simulink model "q_sip_lqr_q8_ip02"  (Simulink 4.00)
settings: Solver=ode4  SolverMode=SingleTasking  StartTime=0.0  StopTime=9999  FixedStep=0.001  RelTol=1e-3  AbsTol=1e-6
values from neighbouring files (symbols this model uses):
  C = eye( 4 )    [d_ip01_2_sip_lqr.m]
  D = zeros( 4, 1 )    [d_ip01_2_sip_lqr.m]
  IC_ALPHA0 = 0    [linearDesign.m]    (also in linearDesign2.m)
undefined symbols (not defined in the file or in its folder): A, ALPHA_LIM_ENABLE, ALPHA_MAX, ALPHA_MIN, B, K, K_CABLE, K_EC, K_EP, simget, VMAX_DAC, VMAX_UPM, wcf, X_LIM_ENABLE, X_MAX, X_MIN, zetaf
libraries: qctools x7, simulink_extras x3
settings Model: LastModifiedBy=julio  LimitDataPoints=off  SimulationMode=external  RTWSystemTargetFile=wincon.tlc  RTWTemplateMakefile=nt_msvc.tmf  RTWMakeCommand=make_wc  ExtModeMexFile=wc_comm  ExtModeArmWhenConnect=off  OptimizeBlockIOStorage=off

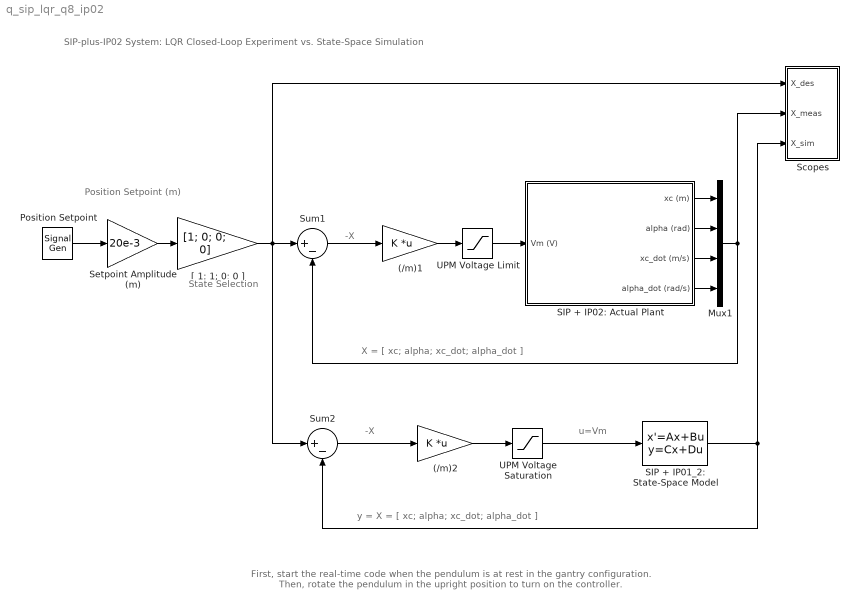
== system q_sip_lqr_q8_ip02 ==
  note: SIP-plus-IP02 System: LQR Closed-Loop
      | Experiment vs. State-Space Simulation
  note: u=Vm
  note: X = [ xc; alpha; xc_dot; alpha_dot ]
  note: -X
  note: -X
  note: State Selection
  note: Position Setpoint (m)
  note: y = X = [ xc; alpha; xc_dot; alpha_dot ]
  note: First, start the real-time code when the pendulum is at rest in the gantry configuration.
      | Then, rotate the pendulum in the upright position to turn on the controller.
  (/m)1 : Gain  Gain=K  Multiplication=Matrix(K*u)  SaturateOnIntegerOverflow=on
  (/m)2 : Gain  Gain=K  Multiplication=Matrix(K*u)  SaturateOnIntegerOverflow=on
  Mux1 : Mux  Inputs=4
  Position Setpoint : SignalGenerator  WaveForm=square  Amplitude=1  Frequency=0.2  Units=Hertz
  SIP + IP01_2: State-Space Model : StateSpace  A=A  B=B  C=C  D=D  X0=[ 0; IC_ALPHA0; 0; 0 ]  AbsoluteTolerance=auto  Realization=auto
  SIP + IP02: Actual Plant : Subsystem
      settings: RTWFcnNameOpts=Auto  RTWFileNameOpts=Auto
  Scopes : Subsystem
      settings: RTWFcnNameOpts=Auto  RTWFileNameOpts=Auto
  Setpoint Amplitude (m) : Gain  Gain=20e-3  Multiplication=Element-wise(K.*u)  SaturateOnIntegerOverflow=on
  Sum1 : Sum  Inputs=|+-  SaturateOnIntegerOverflow=on
  Sum2 : Sum  Inputs=|+-  SaturateOnIntegerOverflow=on
  UPM Voltage Limit : Saturate  UpperLimit=VMAX_UPM  LowerLimit=- VMAX_UPM  LinearizeAsGain=on
  UPM Voltage Saturation : Saturate  UpperLimit=VMAX_UPM  LowerLimit=- VMAX_UPM  LinearizeAsGain=on
  "[ 1; 1; 0; 0 ]" : Gain  Gain=[1; 0; 0; 0]  Multiplication=Element-wise(K.*u)  SaturateOnIntegerOverflow=on
  wires:
  UPM Voltage Limit/1 -> SIP + IP02: Actual Plant/1(Vm (V))
  SIP + IP02: Actual Plant/1(xc (m)) -> Mux1/1
  SIP + IP02: Actual Plant/2(alpha (rad)) -> Mux1/2
  SIP + IP02: Actual Plant/4(alpha_dot (rad/s)) -> Mux1/4
  UPM Voltage Saturation/1 -> SIP + IP01_2: State-Space Model/1
  (/m)2/1 -> UPM Voltage Saturation/1
  Sum2/1 -> (/m)2/1
  "[ 1; 1; 0; 0 ]"/1 -> Sum1/1, Scopes/1(X_des), Sum2/1
  Mux1/1 -> Scopes/2(X_meas), Sum1/2
  SIP + IP01_2: State-Space Model/1 -> Scopes/3(X_sim), Sum2/2
  SIP + IP02: Actual Plant/3(xc_dot (m/s)) -> Mux1/3
  Position Setpoint/1 -> Setpoint Amplitude (m)/1
  Setpoint Amplitude (m)/1 -> "[ 1; 1; 0; 0 ]"/1
  Sum1/1 -> (/m)1/1
  (/m)1/1 -> UPM Voltage Limit/1

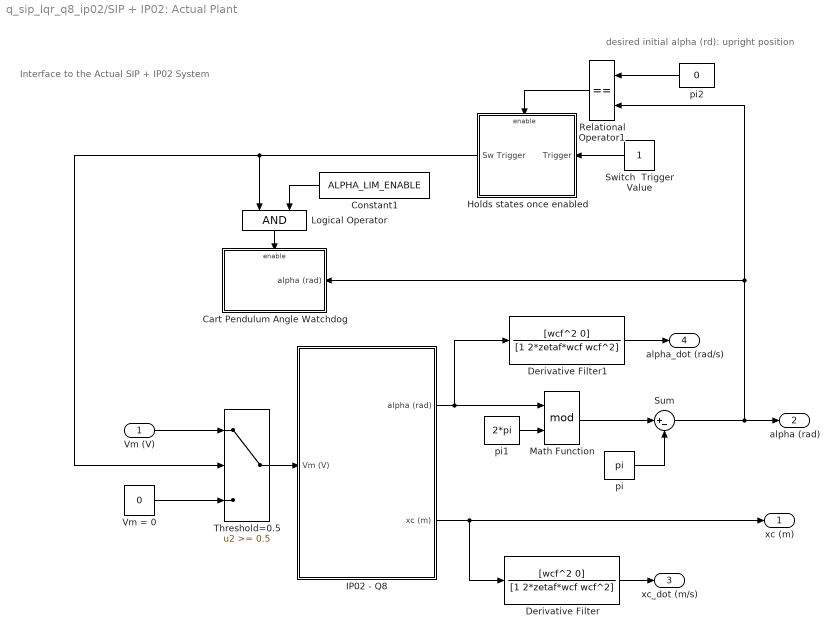
== system q_sip_lqr_q8_ip02/SIP + IP02: Actual Plant ==
  note: Interface to the Actual
      | SIP + IP02 System
  note: desired initial alpha (rd):
      | upright position
  Vm (V) : Inport  Port=1  LatchInput=off
  Cart Pendulum Angle Watchdog : Subsystem  Orientation=left  TreatAsAtomicUnit=on
      settings: RTWFcnNameOpts=Auto  RTWFileNameOpts=Auto
  Constant1 : Constant  Orientation=left  Value=ALPHA_LIM_ENABLE
  Derivative Filter : TransferFcn  Numerator=[wcf^2 0]  Denominator=[1 2*zetaf*wcf wcf^2]  AbsoluteTolerance=auto  Realization=auto
  Derivative Filter1 : TransferFcn  Numerator=[wcf^2 0]  Denominator=[1 2*zetaf*wcf wcf^2]  AbsoluteTolerance=auto  Realization=auto
  Holds states once enabled : Subsystem  Orientation=left  TreatAsAtomicUnit=on
      settings: RTWFcnNameOpts=Auto  RTWFileNameOpts=Auto
  IP02 - Q8 : Subsystem
      settings: RTWFcnNameOpts=Auto  RTWFileNameOpts=Auto
  Logical Operator : Logic  Orientation=down  Operator=AND  Inputs=2
  Math Function : Math  Operator=mod  OutputSignalType=auto
  Relational Operator1 : RelationalOperator  Orientation=left  Operator===
  Sum : Sum  Inputs=|+-  SaturateOnIntegerOverflow=on
  Switch  Trigger Value : Constant  Orientation=left  Value=1
  Threshold=0.5 : Switch  Threshold=0.5
  Vm = 0 : Constant  Value=0
  pi : Constant  Value=pi
  pi1 : Constant  Value=2*pi
  pi2 : Constant  Orientation=left  Value=0
  xc (m) : Outport  Port=1  InitialOutput=0
  alpha (rad) : Outport  Port=2  InitialOutput=0
  xc_dot (m/s) : Outport  Port=3  InitialOutput=0
  alpha_dot (rad/s) : Outport  Port=4  InitialOutput=0
  wires:
  IP02 - Q8/2(xc (m)) -> xc (m)/1, Derivative Filter/1
  Derivative Filter1/1 -> alpha_dot (rad/s)/1
  IP02 - Q8/1(alpha (rad)) -> Derivative Filter1/1, Math Function/1
  Derivative Filter/1 -> xc_dot (m/s)/1
  pi1/1 -> Math Function/2
  pi2/1 -> Relational Operator1/1
  Switch  Trigger Value/1 -> Holds states once enabled/1(Trigger)
  Relational Operator1/1 -> Holds states once enabled/Enable
  Threshold=0.5/1 -> IP02 - Q8/1(Vm (V))
  Holds states once enabled/1(Sw Trigger) -> Threshold=0.5/2, Logical Operator/1
  Vm (V)/1 -> Threshold=0.5/1
  Vm = 0/1 -> Threshold=0.5/3
  pi/1 -> Sum/2
  Sum/1 -> alpha (rad)/1, Relational Operator1/2, Cart Pendulum Angle Watchdog/1(alpha (rad))
  Math Function/1 -> Sum/1
  Logical Operator/1 -> Cart Pendulum Angle Watchdog/Enable
  Constant1/1 -> Logical Operator/2

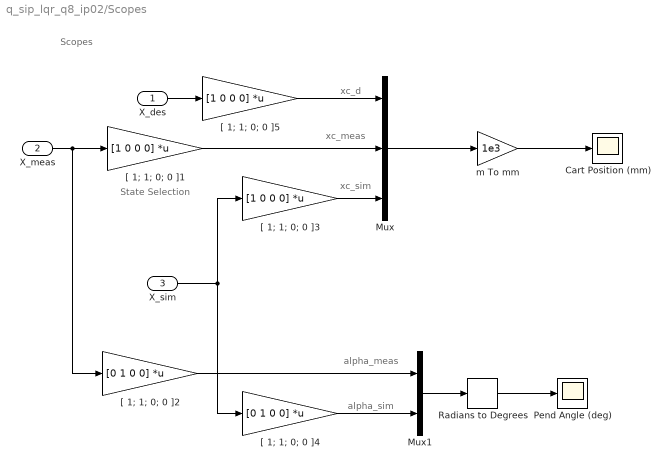
== system q_sip_lqr_q8_ip02/Scopes ==
  note: xc_meas
  note: State Selection
  note: alpha_meas
  note: alpha_sim
  note: xc_sim
  note: xc_d
  note: Scopes
  X_des : Inport  Port=1  LatchInput=off
  X_meas : Inport  Port=2  LatchInput=off
  X_sim : Inport  Port=3  LatchInput=off
  Cart Position (mm) : Scope
      settings: TickLabels=on  TimeRange=1.000000  YMin=-250  YMax=250  SaveToWorkspace=off  DataFormat=Array  LimitDataPoints=on  MaxDataPoints=5000
  Mux : Mux  Inputs=3
  Mux1 : Mux  Inputs=2
  Pend Angle (deg) : Scope
      settings: TickLabels=on  TimeRange=1.000000  YMin=-250  YMax=250  SaveToWorkspace=off  SaveName=ScopeData  DataFormat=Array  LimitDataPoints=on  MaxDataPoints=5000
  Radians to Degrees : simulink_extras/Transformations/Radians to Degrees
  "[ 1; 1; 0; 0 ]1" : Gain  Gain=[1 0 0 0]  Multiplication=Matrix(K*u)  SaturateOnIntegerOverflow=on
  "[ 1; 1; 0; 0 ]2" : Gain  Gain=[0 1 0 0]  Multiplication=Matrix(K*u)  SaturateOnIntegerOverflow=on
  "[ 1; 1; 0; 0 ]3" : Gain  Gain=[1 0 0 0]  Multiplication=Matrix(K*u)  SaturateOnIntegerOverflow=on
  "[ 1; 1; 0; 0 ]4" : Gain  Gain=[0 1 0 0]  Multiplication=Matrix(K*u)  SaturateOnIntegerOverflow=on
  "[ 1; 1; 0; 0 ]5" : Gain  Gain=[1 0 0 0]  Multiplication=Matrix(K*u)  SaturateOnIntegerOverflow=on
  m To mm : Gain  Gain=1e3  Multiplication=Element-wise(K.*u)  SaturateOnIntegerOverflow=on
  wires:
  Mux/1 -> m To mm/1
  m To mm/1 -> Cart Position (mm)/1
  "[ 1; 1; 0; 0 ]1"/1 -> Mux/2
  X_des/1 -> "[ 1; 1; 0; 0 ]5"/1
  X_meas/1 -> "[ 1; 1; 0; 0 ]1"/1, "[ 1; 1; 0; 0 ]2"/1
  Mux1/1 -> Radians to Degrees/1
  Radians to Degrees/1 -> Pend Angle (deg)/1
  X_sim/1 -> "[ 1; 1; 0; 0 ]3"/1, "[ 1; 1; 0; 0 ]4"/1
  "[ 1; 1; 0; 0 ]3"/1 -> Mux/3
  "[ 1; 1; 0; 0 ]5"/1 -> Mux/1
  "[ 1; 1; 0; 0 ]2"/1 -> Mux1/1
  "[ 1; 1; 0; 0 ]4"/1 -> Mux1/2

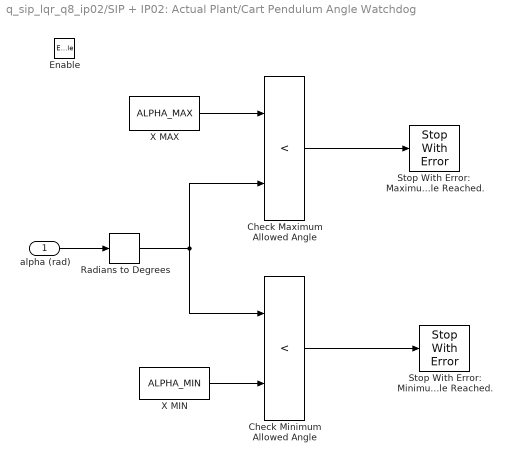
== system q_sip_lqr_q8_ip02/SIP + IP02: Actual Plant/Cart Pendulum Angle Watchdog ==
  alpha (rad) : Inport  Port=1  LatchInput=off
  Enable : EnablePort
  Check Maximum Allowed Angle : RelationalOperator  Operator=<
  Check Minimum Allowed Angle : RelationalOperator  Operator=<
  Radians to Degrees : simulink_extras/Transformations/Radians to Degrees
  Stop With Error: Minimum Angle Reached. : qctools/Extra Sinks/Stop With Error  errMsg=Minimum Angle Limit Reached.
  Stop With Error:  Maximum Angle Reached. : qctools/Extra Sinks/Stop With Error  errMsg=Maximum Angle Limit Reached.
  X MAX : Constant  Value=ALPHA_MAX
  X MIN : Constant  Value=ALPHA_MIN
  wires:
  X MAX/1 -> Check Maximum Allowed Angle/1
  Check Minimum Allowed Angle/1 -> Stop With Error: Minimum Angle Reached./1
  X MIN/1 -> Check Minimum Allowed Angle/2
  alpha (rad)/1 -> Radians to Degrees/1
  Check Maximum Allowed Angle/1 -> Stop With Error:  Maximum Angle Reached./1
  Radians to Degrees/1 -> Check Maximum Allowed Angle/2, Check Minimum Allowed Angle/1

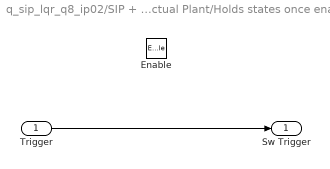
== system q_sip_lqr_q8_ip02/SIP + IP02: Actual Plant/Holds states once enabled ==
  Trigger : Inport  Port=1  LatchInput=off
  Enable : EnablePort
  Sw Trigger : Outport  Port=1  InitialOutput=[0]
  wires:
  Trigger/1 -> Sw Trigger/1

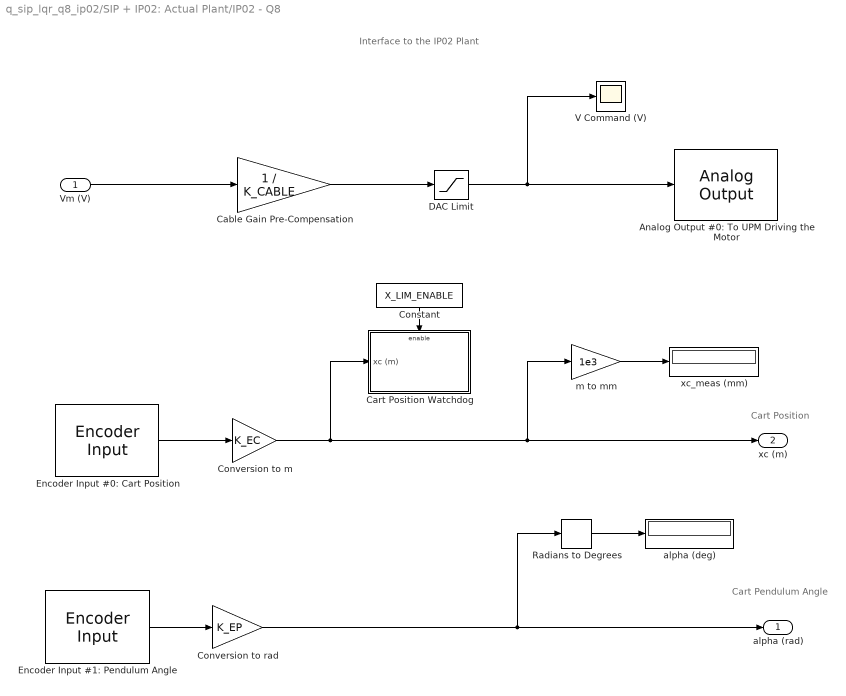
== system q_sip_lqr_q8_ip02/SIP + IP02: Actual Plant/IP02 - Q8 ==
  note: Cart Position
  note: Cart Pendulum Angle
  note: Interface to the IP02 Plant
  Vm (V) : Inport  Port=1  LatchInput=off
  Analog Output #0: To UPM Driving the Motor : qctools/Quanser Consulting Q8 Series/Analog Output  boardNumber=0  channels=0  modesVect=0  rangesVect=10  initialVect=0  finalVect=0  sampleTime=-1  inputVolts=on  simulationOutput=off
  Cable Gain Pre-Compensation : Gain  Gain=1 / K_CABLE  Multiplication=Element-wise(K.*u)  SaturateOnIntegerOverflow=on
  Cart Position Watchdog : Subsystem  TreatAsAtomicUnit=on
      settings: RTWFcnNameOpts=Auto  RTWFileNameOpts=Auto
  Constant : Constant  Orientation=down  Value=X_LIM_ENABLE
  Conversion to m : Gain  Gain=K_EC  Multiplication=Element-wise(K.*u)  SaturateOnIntegerOverflow=on
  Conversion to rad : Gain  Gain=K_EP  Multiplication=Element-wise(K.*u)  SaturateOnIntegerOverflow=on
  DAC Limit : Saturate  UpperLimit=VMAX_DAC  LowerLimit=- VMAX_DAC  LinearizeAsGain=on
  Encoder Input #0: Cart Position : qctools/Quanser Consulting Q8 Series/Encoder Input  boardNumber=0  channels=0  initial=0  sampleTime=simget(bdroot,'FixedStep')  quadratureStr=4X  modeStr=Normal  flagString=FLG1 is IDX and FLG2 is E  prescale=1  frequency=16666666.6667  bcd=off  enableIndex=on  indexPolarity=on  reloadOnIndex=off  simulationInput=off
  Encoder Input #1: Pendulum Angle : qctools/Quanser Consulting Q8 Series/Encoder Input  boardNumber=0  channels=1  initial=0  sampleTime=simget(bdroot,'FixedStep')  quadratureStr=4X  modeStr=Normal  flagString=FLG1 is IDX and FLG2 is E  prescale=1  frequency=16666666.6667  bcd=off  enableIndex=on  indexPolarity=on  reloadOnIndex=off  simulationInput=off
  Radians to Degrees : simulink_extras/Transformations/Radians to Degrees
  V Command (V) : Scope
      settings: TickLabels=on  TimeRange=1.000000  YMin=-1  YMax=1  SaveToWorkspace=off  SaveName=ScopeData3  DataFormat=Array  LimitDataPoints=on  MaxDataPoints=5000
  alpha (deg) : Display
      settings: Format=short
  m to mm : Gain  Gain=1e3  Multiplication=Element-wise(K.*u)  SaturateOnIntegerOverflow=on
  xc_meas (mm) : Display
      settings: Format=short
  alpha (rad) : Outport  Port=1  InitialOutput=0
  xc (m) : Outport  Port=2  InitialOutput=0
  wires:
  DAC Limit/1 -> V Command (V)/1, Analog Output #0: To UPM Driving the Motor/1
  Constant/1 -> Cart Position Watchdog/Enable
  Conversion to rad/1 -> alpha (rad)/1, Radians to Degrees/1
  Radians to Degrees/1 -> alpha (deg)/1
  Encoder Input #1: Pendulum Angle/1 -> Conversion to rad/1
  m to mm/1 -> xc_meas (mm)/1
  Cable Gain Pre-Compensation/1 -> DAC Limit/1
  Conversion to m/1 -> m to mm/1, xc (m)/1, Cart Position Watchdog/1(xc (m))
  Vm (V)/1 -> Cable Gain Pre-Compensation/1
  Encoder Input #0: Cart Position/1 -> Conversion to m/1

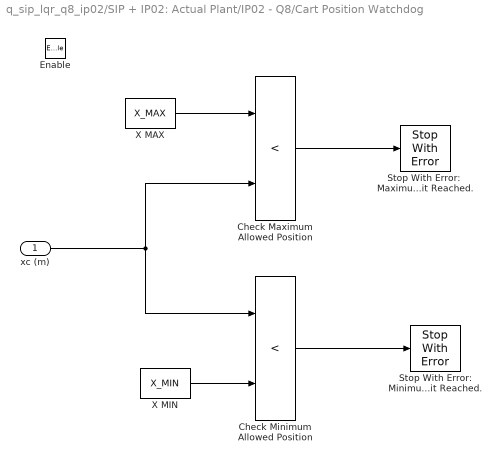
== system q_sip_lqr_q8_ip02/SIP + IP02: Actual Plant/IP02 - Q8/Cart Position Watchdog ==
  xc (m) : Inport  Port=1  LatchInput=off
  Enable : EnablePort
  Check Maximum Allowed Position : RelationalOperator  Operator=<
  Check Minimum Allowed Position : RelationalOperator  Operator=<
  Stop With Error: Minimum Limit Reached. : qctools/Extra Sinks/Stop With Error  errMsg=Minimum Position Limit reached.
  Stop With Error:  Maximum Limit Reached. : qctools/Extra Sinks/Stop With Error  errMsg=Maximum Position Limit reached.
  X MAX : Constant  Value=X_MAX
  X MIN : Constant  Value=X_MIN
  wires:
  X MAX/1 -> Check Maximum Allowed Position/1
  Check Minimum Allowed Position/1 -> Stop With Error: Minimum Limit Reached./1
  X MIN/1 -> Check Minimum Allowed Position/2
  xc (m)/1 -> Check Maximum Allowed Position/2, Check Minimum Allowed Position/1
  Check Maximum Allowed Position/1 -> Stop With Error:  Maximum Limit Reached./1
